simulink model "scope_model_lab_1"  (R2021b)
settings: Solver=VariableStepAuto  StartTime=0.0  StopTime=5  MaxStep=1e-3  RelTol=1e-3
values from neighbouring files (symbols this model uses):
  a11 = -3    [script_lab_1.m]
  a12 = -2    [script_lab_1.m]
  a21 = -5    [script_lab_1.m]
  a22 = -6    [script_lab_1.m]
  b11 = 3    [script_lab_1.m]
  b12 = 7    [script_lab_1.m]
undefined symbols (not defined in the file or in its folder): u1, u2
settings Model: Creator=79159  LastModifiedBy=79159

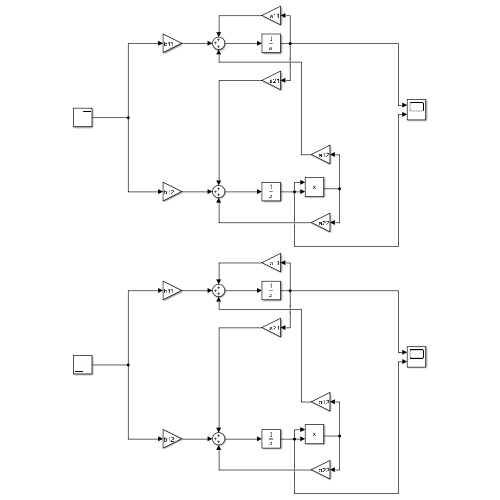
[thumbnail: Simulink's stored preview of the top-level diagram]
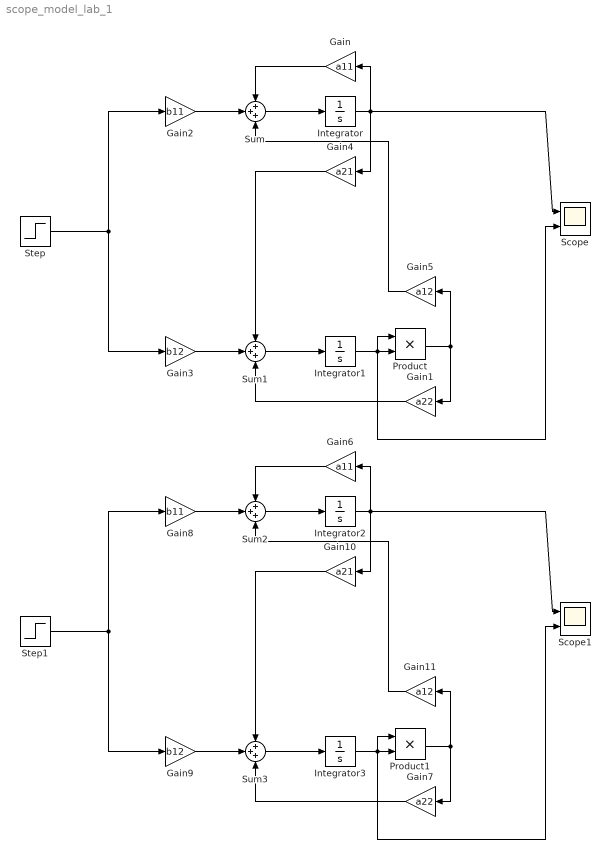
== system scope_model_lab_1 ==
  Gain : Gain  Gain=a11
  Gain1 : Gain  Gain=a22
  Gain10 : Gain  Gain=a21
  Gain11 : Gain  Gain=a12
  Gain2 : Gain  Gain=b11
  Gain3 : Gain  Gain=b12
  Gain4 : Gain  Gain=a21
  Gain5 : Gain  Gain=a12
  Gain6 : Gain  Gain=a11
  Gain7 : Gain  Gain=a22
  Gain8 : Gain  Gain=b11
  Gain9 : Gain  Gain=b12
  Integrator{,1..3} (4 alike) : Integrator
  Product : Product
  Product1 : Product
  Scope : Scope  NumInputPorts=2
  Scope1 : Scope  NumInputPorts=2
  Step : Step  Time=0  After=u1  SampleTime=0
  Step1 : Step  Time=0  After=u2  SampleTime=0
  Sum{,1..3} (4 alike) : Sum  Inputs=+++
  wires:
  Integrator/1 -> Gain4/1, Scope/1, Gain/1
  Sum1/1 -> Integrator1/1
  Sum/1 -> Integrator/1
  Gain3/1 -> Sum1/2
  Gain2/1 -> Sum/2
  Step/1 -> Gain2/1, Gain3/1
  Gain/1 -> Sum/1
  Gain4/1 -> Sum1/1
  Gain1/1 -> Sum1/3
  Gain5/1 -> Sum/3
  Integrator1/1 -> Product/1, Scope/2, Product/2
  Product/1 -> Gain5/1, Gain1/1
  Product1/1 -> Gain7/1, Gain11/1
  Integrator3/1 -> Product1/2, Scope1/2, Product1/1
  Gain11/1 -> Sum2/3
  Gain7/1 -> Sum3/3
  Gain10/1 -> Sum3/1
  Gain6/1 -> Sum2/1
  Step1/1 -> Gain9/1, Gain8/1
  Gain8/1 -> Sum2/2
  Gain9/1 -> Sum3/2
  Sum2/1 -> Integrator2/1
  Sum3/1 -> Integrator3/1
  Integrator2/1 -> Gain6/1, Scope1/1, Gain10/1
